simulink model "SOS_ZPK_PIPELINE_STUART_LANDAU_V1"  (R2024a)
settings: Solver=VariableStepAuto  StartTime=0.0  StopTime=10  RelTol=1e-3
undefined symbols (not defined in the file): A, A_K0, A_KPPO, Appo, B, B_K0, B_KPPO, beta, Bppo, C, C_K0, C_KPPO, Cppo, D, D_K0, D_KPPO, Dppo, mu_target, Ts, w, x0
settings Model: Creator=Personal  LastModifiedBy=Personal

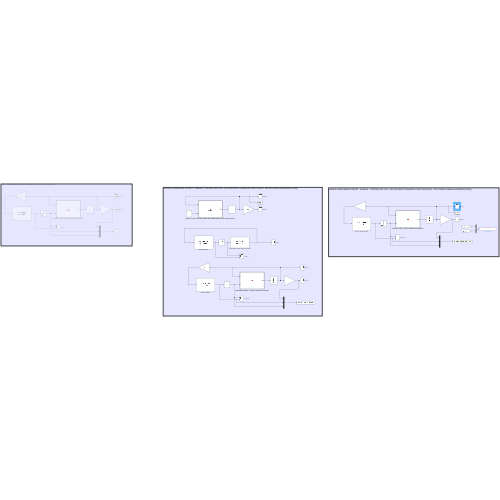
[thumbnail: Simulink's stored preview of the top-level diagram]
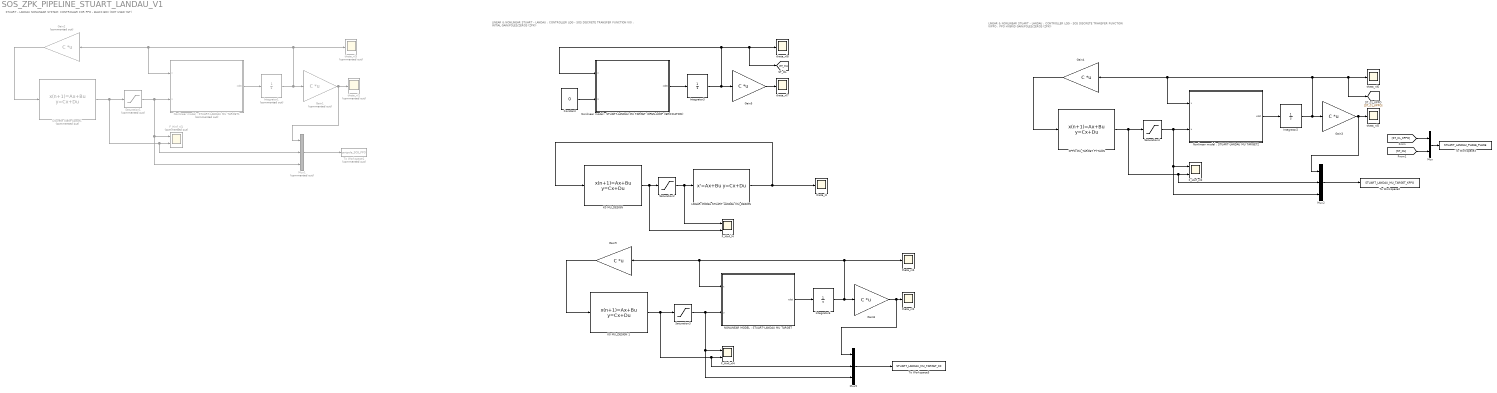
== system SOS_ZPK_PIPELINE_STUART_LANDAU_V1 ==
  note: STUART - LANDAU NONLINEAR SYSTEM: CONTROLLER FOR PPO - BLACK BOX (NOT USED YET)
  note: LINEAR & NONLINEAR STUART - LANDAU : CONTROLLER LQG - SOS DISCRETE TRANSFER FUNCTION (KPPO : PPO HYBRID GAIN/POLES/ZEROS (ZPK))
  note: LINEAR & NONLINEAR STUART - LANDAU : CONTROLLER LQG - SOS DISCRETE TRANSFER FUNCTION (K0 : INITIAL GAIN/POLES/ZEROS (ZPK))
  Constant : Constant  Value=0
  Discrete State-Space1 : DiscreteStateSpace  Commented=on  A=Appo  B=Bppo  C=Cppo  D=Dppo  InitialCondition=zeros(length(Appo),1)  SampleTime=Ts
  F_Hinf_l4 : Scope  NumInputPorts=2
  F_Hinf_nl1 : Scope  Commented=on  NumInputPorts=2
  F_Hinf_nl2 : Scope  NumInputPorts=2
  F_Hinf_nl4 : Scope  NumInputPorts=2
  Gain1 : Gain  Commented=on  Gain=C  Multiplication=Matrix(K*u)
  Gain2 : Gain  Commented=on  Gain=C  Multiplication=Matrix(K*u)
  Gain{3..5,8..9} (5 alike) : Gain  Gain=C  Multiplication=Matrix(K*u)
  Integrator1 : Integrator  Commented=on  InitialCondition=x0
  Integrator2 : Integrator  InitialCondition=x0
  Integrator3 : Integrator  InitialCondition=x0
  Integrator6 : Integrator  InitialCondition=x0
  "K0 MU_DESIGN " : DiscreteStateSpace  A=A_K0  B=B_K0  C=C_K0  D=D_K0  InitialCondition=zeros(length(A_K0),1)  SampleTime=Ts
  K0 MU_DESIGN 1 : DiscreteStateSpace  A=A_K0  B=B_K0  C=C_K0  D=D_K0  InitialCondition=zeros(length(A_K0),1)  SampleTime=Ts
  KPPO MU_TARGET PYTHON : DiscreteStateSpace  A=A_KPPO  B=B_KPPO  C=C_KPPO  D=D_KPPO  InitialCondition=zeros(length(A_KPPO),1)  SampleTime=Ts
  LINEAR MODEL STUART LANDAU MU_DESIGN : StateSpace  A=A  B=B  C=C  D=D  InitialCondition=x0
  Mux : Mux  Inputs=2
  Mux1 : Mux  Commented=on  Inputs=3
  Mux2 : Mux  Inputs=3
  Mux5 : Mux  Inputs=3
  "NONLINEAR MODEL : STUART-LANDAU MU TARGET" : MATLAB Function  TreatAsAtomicUnit=on
  "Nonlinear model : STUART-LANDAU MU TARGET (OPEN-LOOP VERIFICATION)" : MATLAB Function  TreatAsAtomicUnit=on
  "Nonlinear model : STUART-LANDAU MU TARGET1" : MATLAB Function  Commented=on  TreatAsAtomicUnit=on
  "Nonlinear model : STUART-LANDAU MU TARGET2" : MATLAB Function  TreatAsAtomicUnit=on
  Saturation1 : Saturate  Commented=on  UpperLimit=15  LowerLimit=-15
  Saturation2 : Saturate  UpperLimit=15  LowerLimit=-15
  Saturation3 : Saturate  UpperLimit=15  LowerLimit=-15
  Saturation4 : Saturate  UpperLimit=15  LowerLimit=-15
  To Workspace1 : ToWorkspace  Commented=on  VariableName=cartpole_SOS_PPO  SaveFormat=Timeseries  SampleTime=-1
  To Workspace2 : ToWorkspace  VariableName=STUART_LANDAU_MU_TARGET_KPPO  SaveFormat=Timeseries  SampleTime=-1
  To Workspace3 : ToWorkspace  VariableName=STUART_LANDAU_PHASE_PLANE  SaveFormat=Timeseries  SampleTime=-1
  To Workspace5 : ToWorkspace  VariableName=STUART_LANDAU_MU_TARGET_K0  SaveFormat=Timeseries  SampleTime=-1
  theta_l2 : Scope
  theta_nl1 : Scope  Commented=on
  theta_nl{2,4..8} (6 alike) : Scope
  theta_nl3 : Scope  Commented=on
  wires:
  Mux1/1 -> To Workspace1/1
  Saturation2/1 -> LINEAR MODEL STUART LANDAU MU_DESIGN/1, F_Hinf_l4/1
  Saturation3/1 -> "NONLINEAR MODEL : STUART-LANDAU MU TARGET"/2(u), Mux5/3, F_Hinf_nl4/1
  "Nonlinear model : STUART-LANDAU MU TARGET1"/1(xdot) -> Integrator1/1
  Gain1/1 -> Mux1/1, theta_nl1/1
  Gain2/1 -> Discrete State-Space1/1
  Mux5/1 -> To Workspace5/1
  Saturation1/1 -> "Nonlinear model : STUART-LANDAU MU TARGET1"/2(u), Mux1/3, F_Hinf_nl1/1
  LINEAR MODEL STUART LANDAU MU_DESIGN/1 -> "K0 MU_DESIGN "/1, theta_l2/1
  Integrator1/1 -> Gain1/1, theta_nl3/1, "Nonlinear model : STUART-LANDAU MU TARGET1"/1(x), Gain2/1
  Discrete State-Space1/1 -> F_Hinf_nl1/2, Mux1/2, Saturation1/1
  Integrator6/1 -> Gain8/1, theta_nl4/1, "NONLINEAR MODEL : STUART-LANDAU MU TARGET"/1(x), Gain9/1
  "K0 MU_DESIGN "/1 -> Saturation2/1, F_Hinf_l4/2
  Gain8/1 -> Mux5/1, theta_nl2/1
  "NONLINEAR MODEL : STUART-LANDAU MU TARGET"/1(xdot) -> Integrator6/1
  Gain9/1 -> K0 MU_DESIGN 1/1
  K0 MU_DESIGN 1/1 -> Saturation3/1, F_Hinf_nl4/2, Mux5/2
  Saturation4/1 -> "Nonlinear model : STUART-LANDAU MU TARGET2"/2(u), Mux2/3, F_Hinf_nl2/1
  Integrator2/1 -> Gain3/1, [ST_CL_KPPO], theta_nl6/1, "Nonlinear model : STUART-LANDAU MU TARGET2"/1(x), Gain4/1
  KPPO MU_TARGET PYTHON/1 -> F_Hinf_nl2/2, Mux2/2, Saturation4/1
  "Nonlinear model : STUART-LANDAU MU TARGET2"/1(xdot) -> Integrator2/1
  Gain4/1 -> KPPO MU_TARGET PYTHON/1
  Mux2/1 -> To Workspace2/1
  Gain3/1 -> Mux2/1, theta_nl5/1
  Mux/1 -> To Workspace3/1
  Integrator3/1 -> Gain5/1, [ST_OL], theta_nl8/1, "Nonlinear model : STUART-LANDAU MU TARGET (OPEN-LOOP VERIFICATION)"/1(x)
  "Nonlinear model : STUART-LANDAU MU TARGET (OPEN-LOOP VERIFICATION)"/1(xdot) -> Integrator3/1
  Gain5/1 -> theta_nl7/1
  Constant/1 -> "Nonlinear model : STUART-LANDAU MU TARGET (OPEN-LOOP VERIFICATION)"/2(u)
  [ST_CL_KPPO] -> Mux/1
  [ST_OL] -> Mux/2

== matlab function SOS_ZPK_PIPELINE_STUART_LANDAU_V1/Nonlinear model : STUART-LANDAU MU TARGET2 ==
  data: x input; xdot output; u input; mu_target parameter; w parameter; beta parameter
function xdot = derivatives(x,u, mu_target, w, beta)
%xdot as state-variables vector (includes second and first order dynamics)
% x = [x,y]' (2,1)
%Initial conditions (IC) are given in ODE SOLVER (1/s).
xdot = zeros(2,1);
r2 = x(1)^2 + x(2)^2;
xdot(1) = mu_target*x(1) - w*x(2) - r2*(x(1) - beta*x(2)) + u;
xdot(2) = w*x(1) + mu_target*x(2) - r2*(x(2) + beta*x(1));

== matlab function SOS_ZPK_PIPELINE_STUART_LANDAU_V1/Nonlinear model : STUART-LANDAU MU TARGET1 ==
  data: x input; xdot output; u input; mu_target parameter; w parameter; beta parameter
function xdot = derivatives(x,u, mu_target, w, beta)
%xdot as state-variables vector (includes second and first order dynamics)
% x = [x,y]' (2,1)
%Initial conditions (IC) are given in ODE SOLVER (1/s).
xdot = zeros(2,1);
r2 = x(1)^2 + x(2)^2;
xdot(1) = mu_target*x(1) - w*x(2) - r2*(x(1) - beta*x(2)) + u;
xdot(2) = w*x(1) + mu_target*x(2) - r2*(x(2) + beta*x(1));

== matlab function SOS_ZPK_PIPELINE_STUART_LANDAU_V1/Nonlinear model : STUART-LANDAU MU TARGET (OPEN-LOOP VERIFICATION) ==
  data: x input; xdot output; u input; mu_target parameter; w parameter; beta parameter
function xdot = derivatives(x,u, mu_target, w, beta)
%xdot as state-variables vector (includes second and first order dynamics)
% x = [x,y]' (2,1)
%Initial conditions (IC) are given in ODE SOLVER (1/s).
xdot = zeros(2,1);
r2 = x(1)^2 + x(2)^2;
xdot(1) = mu_target*x(1) - w*x(2) - r2*(x(1) - beta*x(2)) + u;
xdot(2) = w*x(1) + mu_target*x(2) - r2*(x(2) + beta*x(1));

== matlab function SOS_ZPK_PIPELINE_STUART_LANDAU_V1/NONLINEAR MODEL : STUART-LANDAU MU TARGET ==
  data: x input; xdot output; u input; mu_target parameter; w parameter; beta parameter
function xdot = derivatives(x,u, mu_target, w, beta)
%xdot as state-variables vector (includes second and first order dynamics)
% x = [x,y]' (2,1)
%Initial conditions (IC) are given in ODE SOLVER (1/s).
xdot = zeros(2,1);
r2 = x(1)^2 + x(2)^2;
xdot(1) = mu_target*x(1) - w*x(2) - r2*(x(1) - beta*x(2)) + u;
xdot(2) = w*x(1) + mu_target*x(2) - r2*(x(2) + beta*x(1));
